simulink model "HybridPlant"  (R2018b)
settings: Solver=VariableStepAuto  StartTime=0.0  StopTime=t_sim  RelTol=1e-3
undefined symbols (not defined in the file or in its folder): Amb, Batt, Lo, Pv, Wt
settings Model: Creator=Pedro  LastModifiedBy=Pedro

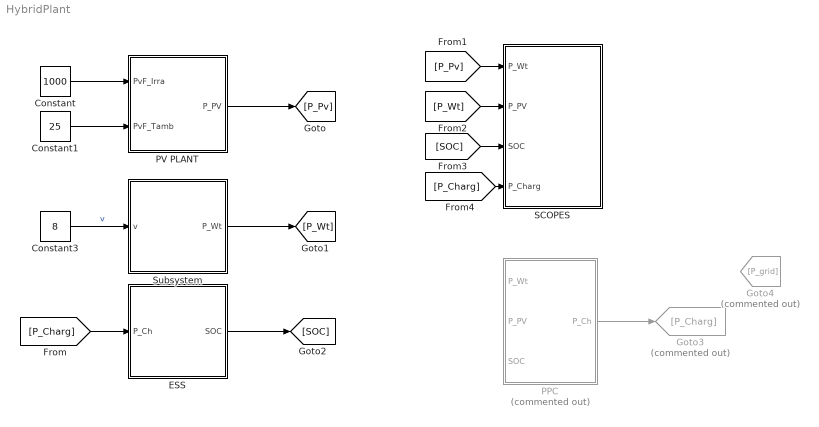
== system HybridPlant ==
  Constant : Constant  Value=1000
  Constant1 : Constant  Value=25
  Constant3 : Constant  Value=8
  ESS : Subsystem
  Goto3 : Goto  Commented=on  GotoTag=P_Charg
  Goto4 : Goto  Commented=on  GotoTag=P_grid
  PPC : Subsystem  Commented=on
  PV PLANT : Subsystem
  "SCOPES " : Subsystem
  Subsystem : Subsystem
  wires:
  PV PLANT/1(P_PV) -> [P_Pv]
  Constant/1 -> PV PLANT/1(PvF_Irra)
  Constant1/1 -> PV PLANT/2(PvF_Tamb)
  Constant3/1 -> Subsystem/1(v)  "v"
  Subsystem/1(P_Wt) -> [P_Wt]
  [P_Charg] -> ESS/1(P_Ch)
  ESS/1(SOC) -> [SOC]
  [P_Pv] -> "SCOPES "/1(P_Wt)
  [P_Wt] -> "SCOPES "/2(P_PV)
  [SOC] -> "SCOPES "/3(SOC)
  PPC/1(P_Ch) -> Goto3/1
  [P_Charg] -> "SCOPES "/4("P_Charg ")

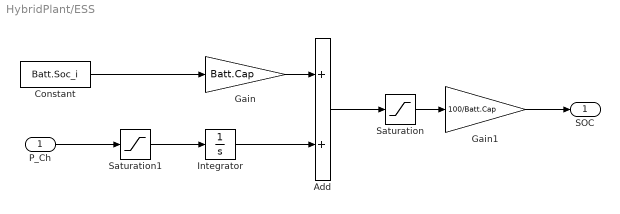
== system HybridPlant/ESS ==
  P_Ch : Inport
  Add : Sum
  Constant : Constant  Value=Batt.Soc_i
  Gain : Gain  Gain=Batt.Cap
  Gain1 : Gain  Gain=100/Batt.Cap
  Integrator : Integrator
  Saturation : Saturate  UpperLimit=Batt.Cap  LowerLimit=0
  Saturation1 : Saturate  UpperLimit=Batt.Pmax  LowerLimit=-Batt.Pmax
  SOC : Outport
  wires:
  Saturation/1 -> Gain1/1
  Gain/1 -> Add/1
  Integrator/1 -> Add/2
  Add/1 -> Saturation/1
  Saturation1/1 -> Integrator/1
  Constant/1 -> Gain/1
  P_Ch/1 -> Saturation1/1
  Gain1/1 -> SOC/1

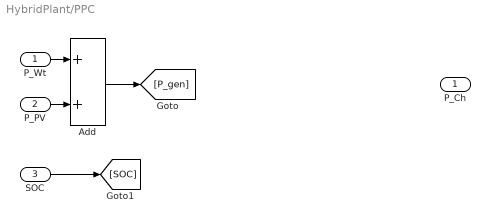
== system HybridPlant/PPC ==
  P_Wt : Inport
  P_PV : Inport  Port=2
  SOC : Inport  Port=3
  Add : Sum
  P_Ch : Outport
  wires:
  ? -> P_Ch/1
  P_Wt/1 -> Add/1
  P_PV/1 -> Add/2
  Add/1 -> [P_gen]
  SOC/1 -> [SOC]

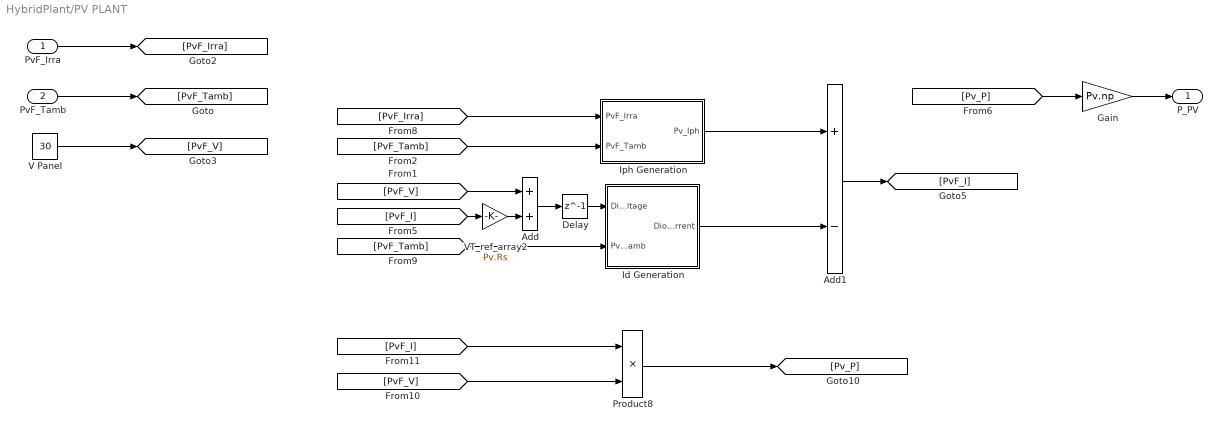
== system HybridPlant/PV PLANT ==
  PvF_Irra : Inport
  PvF_Tamb : Inport  Port=2
  Add : Sum
  Add1 : Sum  Inputs=+-
  Delay : Delay  DelayLength=1
  Gain : Gain  Gain=Pv.np
  Id Generation : Subsystem
  Iph Generation : Subsystem
  Product8 : Product  Inputs=**  RndMeth=Zero
  V Panel : Constant  Value=30
  VT_ref_array2 : Gain  Gain=Pv.Rs
  P_PV : Outport
  wires:
  Delay/1 -> Id Generation/1(Diode Voltage)
  Iph Generation/1(Pv_Iph) -> Add1/1
  Add1/1 -> [PvF_I]
  PvF_Tamb/1 -> [PvF_Tamb]
  PvF_Irra/1 -> [PvF_Irra]
  Add/1 -> Delay/1
  Id Generation/1(Diode Current) -> Add1/2
  V Panel/1 -> [PvF_V]
  VT_ref_array2/1 -> Add/2
  Product8/1 -> [Pv_P]
  [PvF_V] -> Product8/2
  [PvF_I] -> Product8/1
  [PvF_I] -> VT_ref_array2/1
  [Pv_P] -> Gain/1
  [PvF_V] -> Add/1
  [PvF_Tamb] -> Id Generation/2(PvF_Tamb)
  [PvF_Tamb] -> Iph Generation/2(PvF_Tamb)
  [PvF_Irra] -> Iph Generation/1(PvF_Irra)
  Gain/1 -> P_PV/1

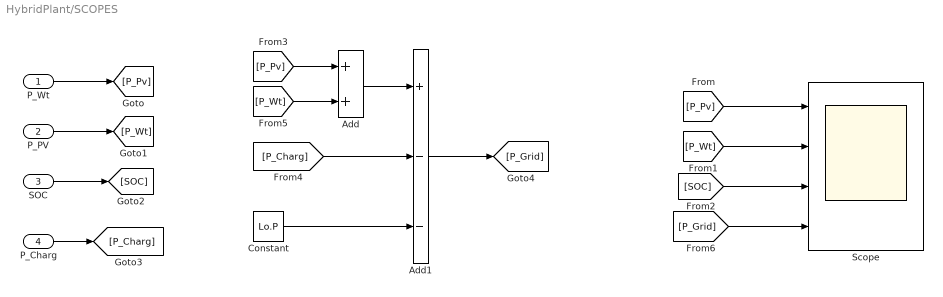
== system HybridPlant/SCOPES  ==
  P_Wt : Inport
  P_PV : Inport  Port=2
  SOC : Inport  Port=3
  "P_Charg " : Inport  Port=4
  Add : Sum
  Add1 : Sum  Inputs=+--
  Constant : Constant  Value=Lo.P
  Scope : Scope  NumInputPorts=4
  wires:
  P_Wt/1 -> [P_Pv]
  P_PV/1 -> [P_Wt]
  SOC/1 -> [SOC]
  [P_Pv] -> Scope/1
  [P_Wt] -> Scope/2
  [SOC] -> Scope/3
  "P_Charg "/1 -> [P_Charg]
  [P_Pv] -> Add/1
  [P_Wt] -> Add/2
  Add/1 -> Add1/1
  [P_Charg] -> Add1/2
  Add1/1 -> [P_Grid]
  Constant/1 -> Add1/3
  [P_Grid] -> Scope/4

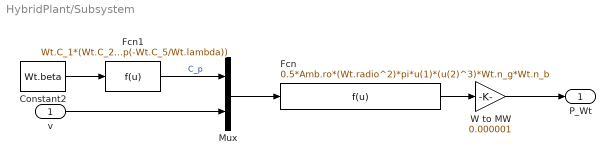
== system HybridPlant/Subsystem ==
  v : Inport
  Constant2 : Constant  Value=Wt.beta
  Fcn : Fcn  Expr=0.5*Amb.ro*(Wt.radio^2)*pi*u(1)*(u(2)^3)*Wt.n_g*Wt.n_b
  Fcn1 : Fcn  Expr=Wt.C_1*(Wt.C_2/Wt.lambda-Wt.C_3*u(1)-Wt.C_7*u(1)^Wt.C_8-Wt.C_4)*(exp(-Wt.C_5/Wt.lambda))
  Mux : Mux  Inputs=2
  W to MW : Gain  Gain=0.000001
  P_Wt : Outport
  wires:
  Constant2/1 -> Fcn1/1
  W to MW/1 -> P_Wt/1
  Fcn1/1 -> Mux/1  "C_p"
  Fcn/1 -> W to MW/1
  Mux/1 -> Fcn/1
  v/1 -> Mux/2

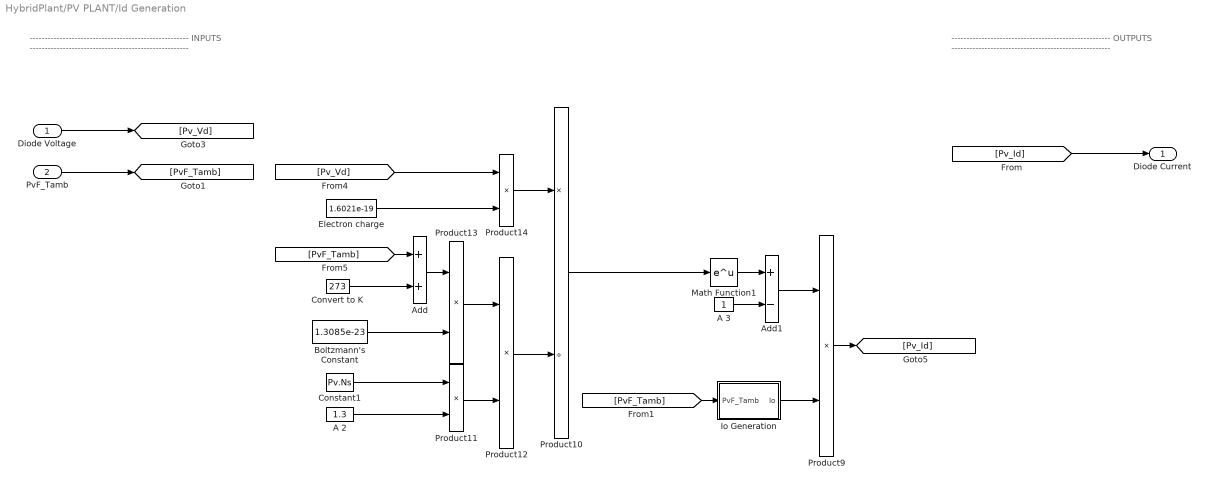
== system HybridPlant/PV PLANT/Id Generation ==
  note: -----------------------------------------------------
      |                          INPUTS
      | -----------------------------------------------------
  note: -----------------------------------------------------
      |                          OUTPUTS
      | -----------------------------------------------------
  Diode Voltage : Inport
  PvF_Tamb : Inport  Port=2
  A 2 : Constant  Value=1.3
  A 3 : Constant
  Add : Sum
  Add1 : Sum  Inputs=+-
  "Boltzmann's Constant " : Constant  Value=1.3085e-23
  Constant1 : Constant  Value=Pv.Ns
  Convert to K : Constant  Value=273
  Electron charge : Constant  Value=1.6021e-19
  Io Generation : Subsystem
  Math Function1 : Math  SaturateOnIntegerOverflow=on
  Product10 : Product  Inputs=*/  RndMeth=Zero
  Product{9,11..14} (5 alike) : Product  Inputs=**  RndMeth=Zero
  Diode Current : Outport
  wires:
  Constant1/1 -> Product11/1
  [PvF_Tamb] -> Io Generation/1(PvF_Tamb)
  "Boltzmann's Constant "/1 -> Product13/2
  Product10/1 -> Math Function1/1
  Add/1 -> Product13/1
  Add1/1 -> Product9/1
  A 3/1 -> Add1/2
  Electron charge/1 -> Product14/2
  Product12/1 -> Product10/2
  A 2/1 -> Product11/2
  Io Generation/1(Io) -> Product9/2
  Product14/1 -> Product10/1
  Product13/1 -> Product12/1
  Product11/1 -> Product12/2
  Convert to K/1 -> Add/2
  Math Function1/1 -> Add1/1
  Product9/1 -> [Pv_Id]
  Diode Voltage/1 -> [Pv_Vd]
  [PvF_Tamb] -> Add/1
  PvF_Tamb/1 -> [PvF_Tamb]
  [Pv_Vd] -> Product14/1
  [Pv_Id] -> Diode Current/1

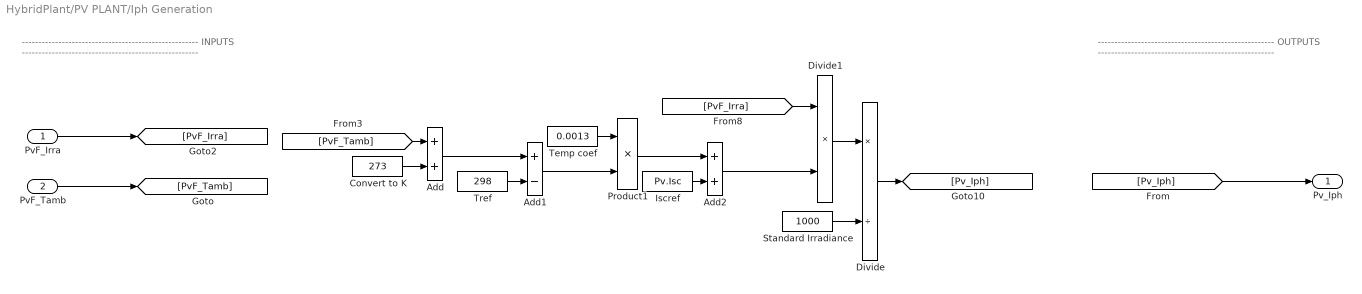
== system HybridPlant/PV PLANT/Iph Generation ==
  note: -----------------------------------------------------
      |                          INPUTS
      | -----------------------------------------------------
  note: -----------------------------------------------------
      |                          OUTPUTS
      | -----------------------------------------------------
  PvF_Irra : Inport
  PvF_Tamb : Inport  Port=2
  Add : Sum
  Add1 : Sum  Inputs=+-
  Add2 : Sum
  "Convert to K " : Constant  Value=273
  Divide : Product  Inputs=*/
  Divide1 : Product  Inputs=**
  Iscref : Constant  Value=Pv.Isc
  Product1 : Product
  Standard Irradiance : Constant  Value=1000
  Temp coef : Constant  Value=0.0013
  "Tref " : Constant  Value=298
  Pv_Iph : Outport
  wires:
  Divide1/1 -> Divide/1
  Divide/1 -> [Pv_Iph]
  Temp coef/1 -> Product1/1
  Product1/1 -> Add2/1
  Standard Irradiance/1 -> Divide/2
  Add/1 -> Add1/1
  Add1/1 -> Product1/2
  [PvF_Tamb] -> Add/1
  [Pv_Iph] -> Pv_Iph/1
  PvF_Tamb/1 -> [PvF_Tamb]
  PvF_Irra/1 -> [PvF_Irra]
  "Convert to K "/1 -> Add/2
  "Tref "/1 -> Add1/2
  Iscref/1 -> Add2/2
  Add2/1 -> Divide1/2
  [PvF_Irra] -> Divide1/1

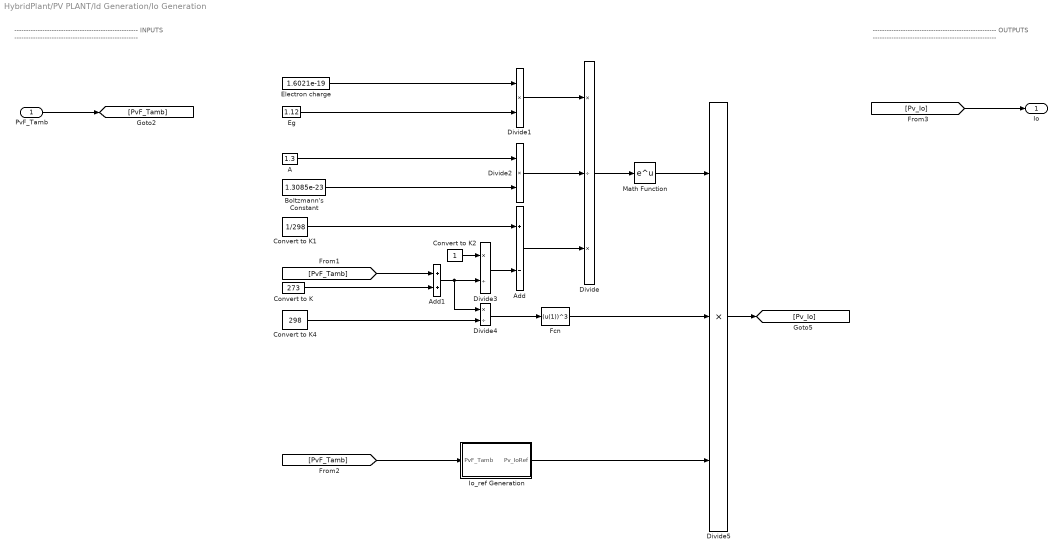
== system HybridPlant/PV PLANT/Id Generation/Io Generation ==
  note: -----------------------------------------------------
      |                          INPUTS
      | -----------------------------------------------------
  note: -----------------------------------------------------
      |                          OUTPUTS
      | -----------------------------------------------------
  PvF_Tamb : Inport
  "A " : Constant  Value=1.3
  Add : Sum  Inputs=+-
  Add1 : Sum
  Boltzmann's Constant : Constant  Value=1.3085e-23
  Convert to K : Constant  Value=273
  Convert to K1 : Constant  Value=1/298
  Convert to K2 : Constant
  Convert to K4 : Constant  Value=298
  Divide : Product  Inputs=*/*
  Divide1 : Product  Inputs=**
  Divide2 : Product  Inputs=**
  Divide3 : Product  Inputs=*/
  Divide4 : Product  Inputs=*/
  Divide5 : Product  Inputs=***
  Eg : Constant  Value=1.12
  Electron charge : Constant  Value=1.6021e-19
  Fcn : Fcn  Expr=(u(1))^3
  Io_ref Generation : Subsystem
  Math Function : Math  SaturateOnIntegerOverflow=on
  Io : Outport
  wires:
  PvF_Tamb/1 -> [PvF_Tamb]
  Add1/1 -> Divide4/1, Divide3/2
  [PvF_Tamb] -> Add1/1
  Convert to K/1 -> Add1/2
  Electron charge/1 -> Divide1/1
  Eg/1 -> Divide1/2
  Divide1/1 -> Divide/1
  "A "/1 -> Divide2/1
  Boltzmann's Constant/1 -> Divide2/2
  Divide2/1 -> Divide/2
  Convert to K1/1 -> Add/1
  Add/1 -> Divide/3
  Convert to K2/1 -> Divide3/1
  Divide3/1 -> Add/2
  Convert to K4/1 -> Divide4/2
  Divide4/1 -> Fcn/1
  Fcn/1 -> Divide5/2
  Io_ref Generation/1(Pv_IoRef) -> Divide5/3
  Divide/1 -> Math Function/1
  Math Function/1 -> Divide5/1
  Divide5/1 -> [Pv_Io]
  [Pv_Io] -> Io/1
  [PvF_Tamb] -> Io_ref Generation/1(PvF_Tamb)

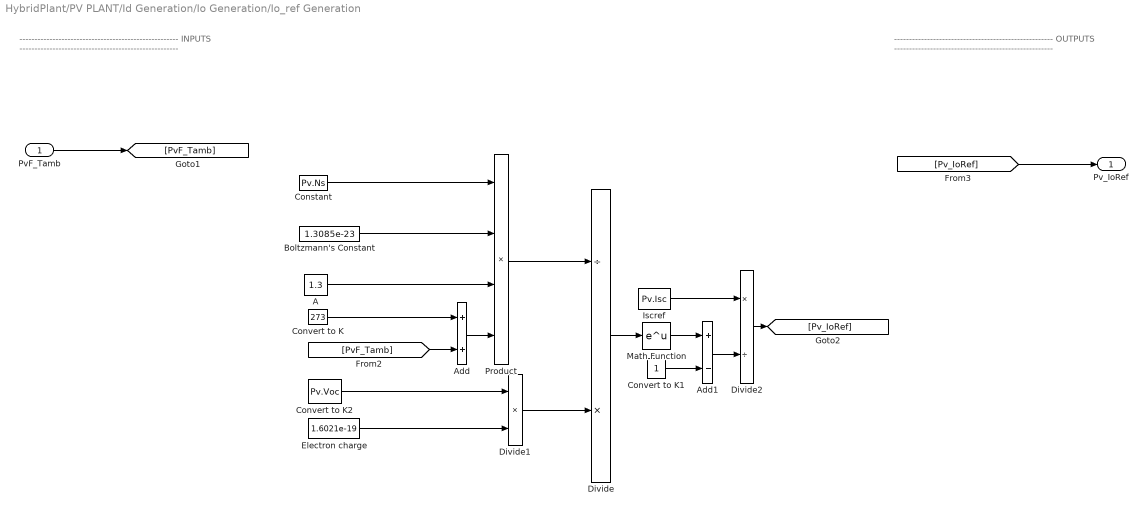
== system HybridPlant/PV PLANT/Id Generation/Io Generation/Io_ref Generation ==
  note: -----------------------------------------------------
      |                          INPUTS
      | -----------------------------------------------------
  note: -----------------------------------------------------
      |                          OUTPUTS
      | -----------------------------------------------------
  PvF_Tamb : Inport
  "A " : Constant  Value=1.3
  Add : Sum
  Add1 : Sum  Inputs=+-
  Boltzmann's Constant : Constant  Value=1.3085e-23
  Constant : Constant  Value=Pv.Ns
  Convert to K : Constant  Value=273
  Convert to K1 : Constant
  Convert to K2 : Constant  Value=Pv.Voc
  Divide : Product  Inputs=/*
  Divide1 : Product  Inputs=**
  Divide2 : Product  Inputs=*/
  Electron charge : Constant  Value=1.6021e-19
  Iscref : Constant  Value=Pv.Isc
  Math Function : Math  SaturateOnIntegerOverflow=on
  Product : Product  Inputs=4
  Pv_IoRef : Outport
  wires:
  PvF_Tamb/1 -> [PvF_Tamb]
  Divide2/1 -> [Pv_IoRef]
  [Pv_IoRef] -> Pv_IoRef/1
  Constant/1 -> Product/1
  Boltzmann's Constant/1 -> Product/2
  "A "/1 -> Product/3
  Convert to K/1 -> Add/1
  Product/1 -> Divide/1
  Divide/1 -> Math Function/1
  Math Function/1 -> Add1/1
  Add1/1 -> Divide2/2
  Iscref/1 -> Divide2/1
  Divide1/1 -> Divide/2
  Electron charge/1 -> Divide1/2
  Convert to K2/1 -> Divide1/1
  [PvF_Tamb] -> Add/2
  Add/1 -> Product/4
  Convert to K1/1 -> Add1/2
